simulink model "ejemplo_simulink"  (R2018a)
settings: Solver=FixedStepDiscrete  StartTime=0.0  StopTime=inf  FixedStep=0.001  RelTol=1e-3  EnableMultiTasking=on
libraries: simulink x2, aerolibanimutils x1
settings Model: Creator=PC  LastModifiedBy=emder
settings OptimizationCC: LifeSpan=inf
settings DebuggingCC: SFUnexpectedBacktrackingDiag=warning  SFNoUnconditionalDefaultTransitionDiag=warning  SFExecutionAtInitializationDiag=none
settings CodeAppCC: StateflowObjectComments=on
settings GRTTargetCC: TargetLangStandard=C89/C90 (ANSI)  GeneratePreprocessorConditionals=Disable all
settings ConfigComp: CovMetricSettings=dw  CovHtmlReporting=on  CovSaveCumulativeToWorkspaceVar=on  CovSaveSingleToWorkspaceVar=on  CovExternalEMLEnable=off

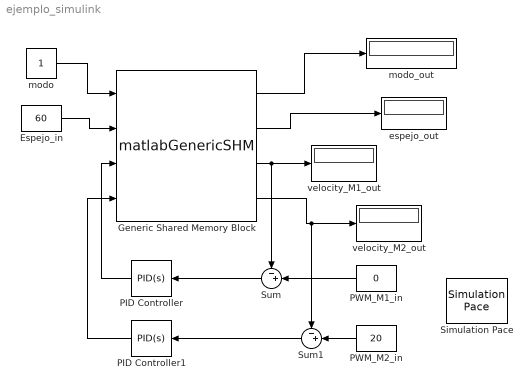
== system ejemplo_simulink ==
  Espejo_in : Constant  Value=60  OutDataTypeStr=single
  Generic Shared Memory Block : S-Function  FunctionName=matlabGenericSHM  Parameters=nombre,dispositivo,vecE,vecS,tipoE,tipoS,ts  SFunctionDeploymentMode=off  EnableBusSupport=off  mask(Generic Share Memory block V2.0){nombre='ARDUINO', dispositivo=1, vecE=[1 1 1 1], vecS=[1 1 1 1], tipoE=['f' 'f' 'f' 'f'], tipoS=['f' 'f' 'f' 'f'], ts=-1}
      mask prompts: nombre "Share Memory base name"; dispositivo "Device Number"; vecE "Sizes input vector"; vecS "Sizes output vector"; tipoE "Data Types Inputs"; tipoS "Data Types Outputs"; ts "Sample Time"
      mask help:
      | This block allows Simulink communication with external processes through shared memory. It works on Unix and Windows.
      | More information in Help.
      mask Help:
      | Share Memory base name (nombre): It's the base string of share memory ej 'robot'
      | Device Number (dispositivo): integer that identifies the device between multiple in use
      | Two shared memorys are created with names:
      | "%name_entrada_%dispositivo" for the device input (writing)
      | "%name_salida_%dispositivo" for the device output (reading)
      | Sizes input vector (vecE)  : array that specify the number of inputs (array dimension) and the inputs size (array values)
      | Sizes output vector  (vecS): array that specify the number of outputs (array dimension) and the outputs size (array values)
      | Data types input(tipoE): char array that specify each input types
      | Data types output (tipoS): char array that specify each output types
      | Allowed types are:
      | ('f'=float, 'd'=double, 'i'=int32, 'c'=char, 'C'= unsigned char, 'I'=unsigned int)
      | Example.
      | Suppose the following parameters:
      | nombre='exampleMemory'
      | dispositivo=10
      | vecE=[3 2 1]
      | vecS=[6 5 7 8]
      | tipoE=['f' 'I' 'c']
      | tipoS=['C' 'i' 'd' 'd']
      | 
      | Two Share Memories are created with names:
      | "exampleMemory_entrada_10" (block input)
      | "exampleMemory_salida_10"  (block output)
      | 3 inputs are created:
      |  1° Dimension 3, type "unsigned char"
      |  2° Dimension 2, type "int"
      |  3° Dimension 1, type "char"
      | 4 outputs are created:
      |  1° Dimension 6, type "float"
      |  2° Dimension 5, type "unsigned int"
      |  3° Dimension 7, type "double"
      |  3° Dimension 8, type "double"
      mask Display: image('shmem.jpg')
  PID Controller : simulink/Continuous/PID Controller  Controller=PID  TimeDomain=Continuous-time  SampleTime=-1  IntegratorMethod=Forward Euler  FilterMethod=Forward Euler  Form=Parallel  UseFilter=on  ControllerParametersSource=internal  P=1  I=0  D=0  N=100  InitialConditionSource=internal  InitialConditionForIntegrator=0  InitialConditionForFilter=0  ExternalReset=none  LimitOutput=off  UpperSaturationLimit=inf  LowerSaturationLimit=-inf  LinearizeAsGain=on  AntiWindupMode=none  Kb=1  TrackingMode=off  Kt=1  PParamMin=[]  PParamMax=[]  IParamMin=[]  IParamMax=[]  DParamMin=[]  DParamMax=[]  NParamMin=[]  NParamMax=[]  KbParamMin=[]  KbParamMax=[]  KtParamMin=[]  KtParamMax=[]  POutMin=[]  POutMax=[]  IOutMin=[]  IOutMax=[]  DOutMin=[]  DOutMax=[]  NOutMin=[]  NOutMax=[]  KbOutMin=[]  KbOutMax=[]  KtOutMin=[]  KtOutMax=[]  IntegratorOutMin=[]  IntegratorOutMax=[]  FilterOutMin=[]  FilterOutMax=[]  SumOutMin=[]  SumOutMax=[]  SumI1OutMin=[]  SumI1OutMax=[]  SumI2OutMin=[]  SumI2OutMax=[]  SumI3OutMin=[]  SumI3OutMax=[]  SumDOutMin=[]  SumDOutMax=[]  SaturationOutMin=[]  SaturationOutMax=[]  IntegratorContinuousStateAttributes=''  IntegratorStateMustResolveToSignalObject=off  IntegratorRTWStateStorageClass=Auto  FilterContinuousStateAttributes=''  FilterStateMustResolveToSignalObject=off  FilterRTWStateStorageClass=Auto  DifferentiatorICPrevScaledInput=0  DifferentiatorOutMin=[]  DifferentiatorOutMax=[]  FilterDiffOutCoefMin=[]  FilterDiffOutCoefMax=[]  SumDenOutMin=[]  SumDenOutMax=[]  SumNumOutMin=[]  SumNumOutMax=[]  ReciprocalOutMin=[]  ReciprocalOutMax=[]  DivideOutMin=[]  DivideOutMax=[]  TunerSelectOption=Transfer Function Based (PID Tuner App)
  PID Controller1 : simulink/Continuous/PID Controller  Controller=PID  TimeDomain=Continuous-time  SampleTime=-1  IntegratorMethod=Forward Euler  FilterMethod=Forward Euler  Form=Parallel  UseFilter=on  ControllerParametersSource=internal  P=1  I=0  D=0  N=100  InitialConditionSource=internal  InitialConditionForIntegrator=0  InitialConditionForFilter=0  ExternalReset=none  LimitOutput=off  UpperSaturationLimit=inf  LowerSaturationLimit=-inf  LinearizeAsGain=on  AntiWindupMode=none  Kb=1  TrackingMode=off  Kt=1  PParamMin=[]  PParamMax=[]  IParamMin=[]  IParamMax=[]  DParamMin=[]  DParamMax=[]  NParamMin=[]  NParamMax=[]  KbParamMin=[]  KbParamMax=[]  KtParamMin=[]  KtParamMax=[]  POutMin=[]  POutMax=[]  IOutMin=[]  IOutMax=[]  DOutMin=[]  DOutMax=[]  NOutMin=[]  NOutMax=[]  KbOutMin=[]  KbOutMax=[]  KtOutMin=[]  KtOutMax=[]  IntegratorOutMin=[]  IntegratorOutMax=[]  FilterOutMin=[]  FilterOutMax=[]  SumOutMin=[]  SumOutMax=[]  SumI1OutMin=[]  SumI1OutMax=[]  SumI2OutMin=[]  SumI2OutMax=[]  SumI3OutMin=[]  SumI3OutMax=[]  SumDOutMin=[]  SumDOutMax=[]  SaturationOutMin=[]  SaturationOutMax=[]  IntegratorContinuousStateAttributes=''  IntegratorStateMustResolveToSignalObject=off  IntegratorRTWStateStorageClass=Auto  FilterContinuousStateAttributes=''  FilterStateMustResolveToSignalObject=off  FilterRTWStateStorageClass=Auto  DifferentiatorICPrevScaledInput=0  DifferentiatorOutMin=[]  DifferentiatorOutMax=[]  FilterDiffOutCoefMin=[]  FilterDiffOutCoefMax=[]  SumDenOutMin=[]  SumDenOutMax=[]  SumNumOutMin=[]  SumNumOutMax=[]  ReciprocalOutMin=[]  ReciprocalOutMax=[]  DivideOutMin=[]  DivideOutMax=[]  TunerSelectOption=Transfer Function Based (PID Tuner App)
  PWM_M1_in : Constant  Value=0  OutDataTypeStr=single
  PWM_M2_in : Constant  Value=20  OutDataTypeStr=single
  Simulation Pace : aerolibanimutils/Simulation Pace  SimulationPace=1  SleepMode=MATLAB Thread  OutputPaceError=off  SampleTime=-1
  Sum : Sum  Inputs=-+|
  Sum1 : Sum  Inputs=-+|
  espejo_out : Display
  modo : Constant  OutDataTypeStr=single  SampleTime=-1
  modo_out : Display
  "velocity_M1_out " : Display
      settings: Decimation=3
  velocity_M2_out : Display
  wires:
  modo/1 -> Generic Shared Memory Block/1
  Generic Shared Memory Block/1 -> modo_out/1
  Generic Shared Memory Block/2 -> espejo_out/1
  Espejo_in/1 -> Generic Shared Memory Block/2
  Generic Shared Memory Block/3 -> Sum/1, "velocity_M1_out "/1
  Generic Shared Memory Block/4 -> Sum1/1, velocity_M2_out/1
  PWM_M1_in/1 -> Sum/2
  PWM_M2_in/1 -> Sum1/2
  Sum/1 -> PID Controller/1
  Sum1/1 -> PID Controller1/1
  PID Controller/1 -> Generic Shared Memory Block/3
  PID Controller1/1 -> Generic Shared Memory Block/4
